simulink model "discrete_and_cont"  (R2019b)
settings: Solver=VariableStepAuto  StartTime=0.0  StopTime=10.0  RelTol=1e-3
undefined symbols (not defined in the file or in its folder): sys, sysd1
settings Model: Creator=Tris  LastModifiedBy=Tris

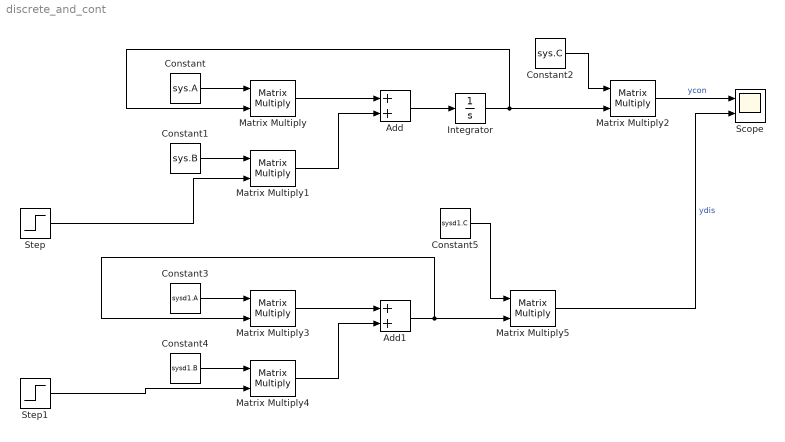
== system discrete_and_cont ==
  Add : Sum
  Add1 : Sum
  Constant : Constant  Value=sys.A
  Constant1 : Constant  Value=sys.B  VectorParams1D=off
  Constant2 : Constant  Value=sys.C  VectorParams1D=off
  Constant3 : Constant  Value=sysd1.A
  Constant4 : Constant  Value=sysd1.B  VectorParams1D=off
  Constant5 : Constant  Value=sysd1.C  VectorParams1D=off
  Integrator : Integrator
  Matrix Multiply{,1..5} (6 alike) : Product  Multiplication=Matrix(*)
  Scope : Scope  NumInputPorts=2
  Step : Step  SampleTime=0  VectorParams1D=off
  Step1 : Step  SampleTime=0  VectorParams1D=off
  wires:
  Matrix Multiply/1 -> Add/1
  Constant/1 -> Matrix Multiply/1
  Add/1 -> Integrator/1
  Integrator/1 -> Matrix Multiply2/2, Matrix Multiply/2
  Matrix Multiply1/1 -> Add/2
  Constant1/1 -> Matrix Multiply1/1
  Step/1 -> Matrix Multiply1/2
  Constant2/1 -> Matrix Multiply2/1
  Matrix Multiply2/1 -> Scope/1  "ycon"
  Matrix Multiply3/1 -> Add1/1
  Matrix Multiply4/1 -> Add1/2
  Constant3/1 -> Matrix Multiply3/1
  Constant4/1 -> Matrix Multiply4/1
  Add1/1 -> Matrix Multiply5/2, Matrix Multiply3/2
  Constant5/1 -> Matrix Multiply5/1
  Matrix Multiply5/1 -> Scope/2  "ydis"
  Step1/1 -> Matrix Multiply4/2
